simulink library "CTRL_LO_ST5"  (R2023b)
settings: Solver=VariableStepAuto  StartTime=0.0  StopTime=10.0  RelTol=1e-3
undefined symbols (not defined in the file): CTRL_LO_p_TqMotLoLim_Nm, CTRL_LO_p_TqMotUpLim_Nm, p_RadWhlDynFr_m, p_RadWhlDynRe_m, p_RatGearFr_na, p_trackFr_m, p_trackRe_m
libraries: slpidlib x4, simulink x1
settings Model: Creator=blatak  LastModifiedBy=blatak

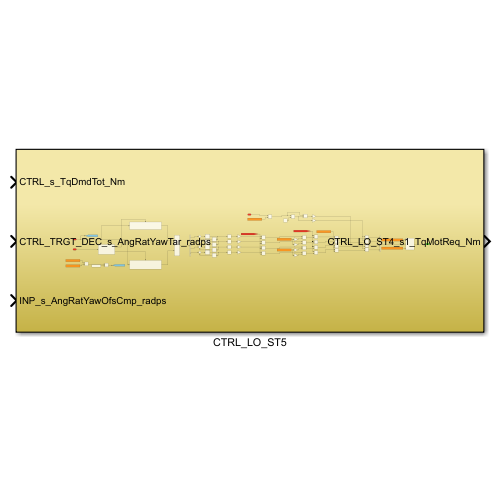
[thumbnail: Simulink's stored preview of the top-level diagram]
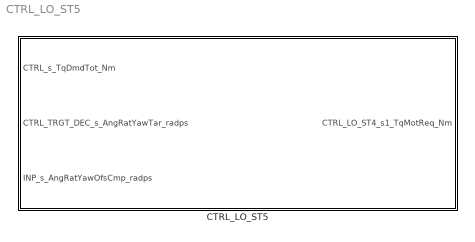
== system CTRL_LO_ST5 ==
  CTRL_LO_ST5 : Subsystem

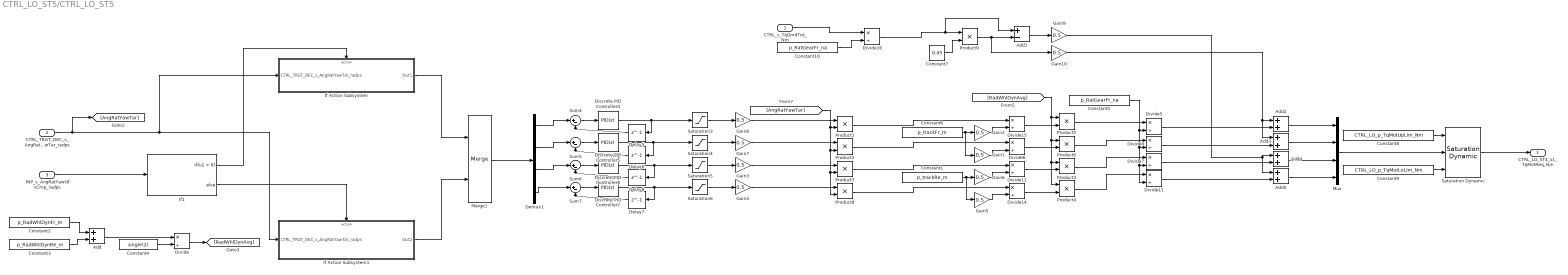
== system CTRL_LO_ST5/CTRL_LO_ST5 ==
  CTRL_s_TqDmdTot_Nm : Inport
  CTRL_TRGT_DEC_s_AngRatYawTar_radps : Inport  Port=2
  INP_s_AngRatYawOfsCmp_radps : Inport  Port=3
  Add{,2..5} (5 alike) : Sum
  Add1 : Sum  Inputs=+-
  Constant1 : Constant  Value=p_trackRe_m
  Constant10 : Constant  Value=p_RatGearFr_na
  Constant2 : Constant  Value=p_RadWhlDynFr_m
  Constant3 : Constant  Value=p_RadWhlDynRe_m
  Constant4 : Constant  Value=single(2)
  Constant5 : Constant  Value=p_RatGearFr_na
  Constant6 : Constant  Value=p_trackFr_m
  Constant7 : Constant  Value=0.45
  Constant8 : Constant  Value=CTRL_LO_p_TqMotUpLim_Nm
  Constant9 : Constant  Value=CTRL_LO_p_TqMotLoLim_Nm
  Delay{5..8} (4 alike) : Delay  DelayLength=1
  Demux1 : Demux
  Discrete PID Controller{4..7} (4 alike) : slpidlib/PID Controller  Controller=PID  Form=Parallel  TimeDomain=Discrete-time  UseExternalTs=off  SampleTime=-1  IntegratorMethod=Forward Euler  FilterMethod=Forward Euler  ControllerParametersSource=internal  P=0.1  I=10  UseKiTs=off  D=0  N=100  UseFilter=on  TunerSelectOption=Transfer Function Based (PID Tuner App)  InitialConditionSource=internal  InitialConditionForIntegrator=0  InitialConditionForFilter=0  DifferentiatorICPrevScaledInput=0  ExternalReset=none  TrackingMode=off  Kt=1  LimitOutput=off  SatLimitsSource=internal  UpperSaturationLimit=inf  LowerSaturationLimit=-inf  LinearizeAsGain=off  AntiWindupMode=none  Kb=1  LimitIntegrator=off  UpperIntegratorSaturationLimit=inf  LowerIntegratorSaturationLimit=-inf  POutMin=[]  POutMax=[]  IOutMin=[]  IOutMax=[]  DOutMin=[]  DOutMax=[]  NOutMin=[]  NOutMax=[]  SumOutMin=[]  SumOutMax=[]  SaturationOutMin=[]  SaturationOutMax=[]  PParamMin=[]  PParamMax=[]  IParamMin=[]  IParamMax=[]  DParamMin=[]  DParamMax=[]  NParamMin=[]  NParamMax=[]  KbParamMin=[]  KbParamMax=[]  KtParamMin=[]  KtParamMax=[]  KbOutMin=[]  KbOutMax=[]  KtOutMin=[]  KtOutMax=[]  IntegratorOutMin=[]  IntegratorOutMax=[]  FilterOutMin=[]  FilterOutMax=[]  SumI1OutMin=[]  SumI1OutMax=[]  SumI2OutMin=[]  SumI2OutMax=[]  SumI3OutMin=[]  SumI3OutMax=[]  SumI4OutMin=[]  SumI4OutMax=[]  SumDOutMin=[]  SumDOutMax=[]  DifferentiatorOutMin=[]  DifferentiatorOutMax=[]  FilterDiffOutCoefMin=[]  FilterDiffOutCoefMax=[]  ReciprocalOutMin=[]  ReciprocalOutMax=[]  SumDenOutMin=[]  SumDenOutMax=[]  SumNumOutMin=[]  SumNumOutMax=[]  DivideOutMin=[]  DivideOutMax=[]  UdiffTsProdOutMin=[]  UdiffTsProdOutMax=[]  NTsProdOutMin=[]  NTsProdOutMax=[]  UintegralTsProdOutMin=[]  UintegralTsProdOutMax=[]  UngainTsProdOutMin=[]  UngainTsProdOutMax=[]  ClampingZeroOutDataTypeStr=Inherit: Inherit via back propagation  ClampingZeroOutMin=[]  ClampingZeroOutMax=[]  FilterDenConstantOutDataTypeStr=Inherit: Inherit via back propagation  FilterDenConstantOutMin=[]  FilterDenConstantOutMax=[]  PCopyOutDataTypeStr=Inherit: Inherit via back propagation  PCopyOutMin=[]  PCopyOutMax=[]  NCopyOutDataTypeStr=Inherit: Inherit via back propagation  NCopyOutMin=[]  NCopyOutMax=[]  IntegratorContinuousStateAttributes=''  IntegratorStateMustResolveToSignalObject=off  IntegratorRTWStateStorageClass=Auto  FilterContinuousStateAttributes=''  FilterStateMustResolveToSignalObject=off  FilterRTWStateStorageClass=Auto  ParallelPVariant=InternalParameters  IdealPVariant=Disabled  IVariant=InternalParameters  DVariant=InternalParameters  IntegratorVariant=Discrete  SatVariant=Disabled  AWVariant=Passthrough  PCopyVariant=Disabled  TRVariant=Disabled  FdbkBlocksVariant=Forward  IdealPFdbkVariant=Disabled  SatFdbkVariant=Disabled  DerivativeFilterVariant=ForwardEulerFilter  NVariant=InternalParameters  NCopyVariant=Disabled  FilterICVariant=InternalICsFilter  IntegratorICVariant=InternalICs  ExternalResetVariant=Disabled  TRSumVariant=Passthrough  SumFdbkVariant=Disabled  SumVariant=Sum_PID  TsampFilterVariant=InternalTs  TsampNgainVariant=Passthrough  TsampIntegralVariant=Disabled_SignalSpec  ExternalSaturationOutDataTypeStr=Inherit: Same as second input
  Divide{,5..8,11..12,14..16} (10 alike) : Product  Inputs=*/
  Gain{1..10} (10 alike) : Gain  Gain=0.5
  If Action Subsystem : Subsystem  TreatAsAtomicUnit=on
  If Action Subsystem1 : Subsystem  TreatAsAtomicUnit=on
  If1 : If
  Merge1 : Merge
  Mux : Mux
  Product{1..9} (9 alike) : Product
  Saturation Dynamic : simulink/Discontinuities/Saturation Dynamic  OutMin=[]  OutMax=[]  OutDataTypeStr=Inherit: Same as second input  OutDataType=fixdt(1, 16)  OutScaling=2^-10  DoSatur=off
  Saturation{3..6} (4 alike) : Saturate  UpperLimit=1  LowerLimit=-1
  Sum{4..7} (4 alike) : Sum  Inputs=|+-
  CTRL_LO_ST4_s1_TqMotReq_Nm : Outport
  wires:
  Constant2/1 -> Add/1
  Constant3/1 -> Add/2
  Add/1 -> Divide/1
  Constant4/1 -> Divide/2
  CTRL_TRGT_DEC_s_AngRatYawTar_radps/1 -> [AngRatYawTar], If Action Subsystem/1(CTRL_TRGT_DEC_s_AngRatYawTar_radps), If Action Subsystem1/1(CTRL_TRGT_DEC_s_AngRatYawTar_radps)
  INP_s_AngRatYawOfsCmp_radps/1 -> If1/1
  If1/1 -> If Action Subsystem/Action
  If1/2 -> If Action Subsystem1/Action
  If Action Subsystem/1(Out1) -> Merge1/1
  If Action Subsystem1/1(Out2) -> Merge1/2
  Divide12/1 -> Product3/2
  Saturation4/1 -> Gain7/1
  Discrete PID Controller6/1 -> Saturation5/1, Delay8/1
  Product7/1 -> Divide12/1
  Demux1/2 -> Sum5/1
  Gain8/1 -> Product1/1
  Product6/1 -> Divide8/1
  Demux1/4 -> Sum7/1
  Gain6/1 -> Divide12/2
  Constant5/1 -> Divide7/2, Divide11/2, Divide8/2, Divide5/2
  Product1/1 -> Divide15/1
  Product2/1 -> Divide6/1
  Demux1/3 -> Sum6/1
  Product8/1 -> Divide14/1
  Saturation3/1 -> Gain8/1
  Gain1/1 -> Divide6/2
  Delay8/1 -> Sum6/2
  Discrete PID Controller5/1 -> Delay6/1, Saturation4/1
  [AngRatYawTar] -> Product7/2, Product8/2, Product2/2, Product1/2
  Discrete PID Controller4/1 -> Saturation3/1, Delay5/1
  Constant1/1 -> Gain5/1, Gain6/1
  Saturation5/1 -> Gain3/1
  Gain7/1 -> Product2/1
  Sum5/1 -> Discrete PID Controller5/1
  Divide6/1 -> Product6/2
  Discrete PID Controller7/1 -> Saturation6/1, Delay7/1
  Sum6/1 -> Discrete PID Controller6/1
  Gain4/1 -> Product8/1
  Demux1/1 -> Sum4/1
  Product5/1 -> Divide5/1
  Delay5/1 -> Sum4/2
  Product3/1 -> Divide7/1
  Product4/1 -> Divide11/1
  Gain2/1 -> Divide15/2
  Delay6/1 -> Sum5/2
  Gain5/1 -> Divide14/2
  Saturation6/1 -> Gain4/1
  Divide14/1 -> Product4/2
  Merge1/1 -> Demux1/1
  Constant6/1 -> Gain1/1, Gain2/1
  Sum7/1 -> Discrete PID Controller7/1
  Delay7/1 -> Sum7/2
  [RadWhlDynAvg] -> Product3/1, Product4/1, Product6/1, Product5/1
  Gain3/1 -> Product7/1
  Divide15/1 -> Product5/2
  Sum4/1 -> Discrete PID Controller4/1
  Divide/1 -> [RadWhlDynAvg]
  CTRL_s_TqDmdTot_Nm/1 -> Divide16/1
  Product9/1 -> Add1/2, Gain10/1
  Gain9/1 -> Add4/1, Add5/1
  Add1/1 -> Gain9/1
  Constant7/1 -> Product9/2
  Divide16/1 -> Product9/1, Add1/1
  Gain10/1 -> Add3/1, Add2/1
  Constant10/1 -> Divide16/2
  Divide5/1 -> Add2/2
  Divide8/1 -> Add3/2
  Divide7/1 -> Add4/2
  Divide11/1 -> Add5/2
  Add5/1 -> Mux/4
  Add4/1 -> Mux/3
  Add3/1 -> Mux/2
  Add2/1 -> Mux/1
  Constant8/1 -> Saturation Dynamic/1
  Constant9/1 -> Saturation Dynamic/3
  Mux/1 -> Saturation Dynamic/2
  Saturation Dynamic/1 -> CTRL_LO_ST4_s1_TqMotReq_Nm/1

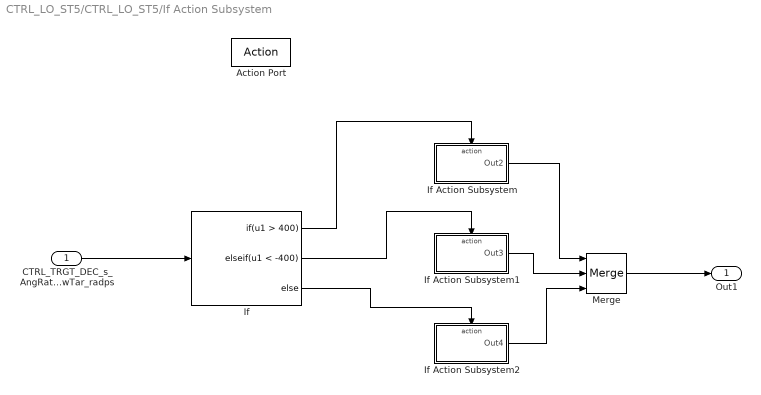
== system CTRL_LO_ST5/CTRL_LO_ST5/If Action Subsystem ==
  CTRL_TRGT_DEC_s_AngRatYawTar_radps : Inport
  Action Port : ActionPort  ActionPortLabel=if(u1 > 0)
  If : If  IfExpression=u1 > 400  ElseIfExpressions=u1 < -400
  If Action Subsystem : Subsystem  TreatAsAtomicUnit=on
  If Action Subsystem1 : Subsystem  TreatAsAtomicUnit=on
  If Action Subsystem2 : Subsystem  TreatAsAtomicUnit=on
  Merge : Merge  Inputs=3
  Out1 : Outport
  wires:
  If Action Subsystem2/1(Out4) -> Merge/3
  CTRL_TRGT_DEC_s_AngRatYawTar_radps/1 -> If/1
  If/2 -> If Action Subsystem1/Action
  If/1 -> If Action Subsystem/Action
  If Action Subsystem1/1(Out3) -> Merge/2
  If/3 -> If Action Subsystem2/Action
  Merge/1 -> Out1/1
  If Action Subsystem/1(Out2) -> Merge/1

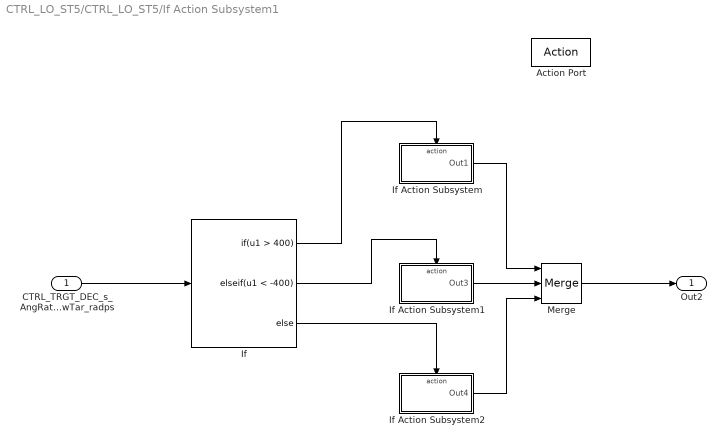
== system CTRL_LO_ST5/CTRL_LO_ST5/If Action Subsystem1 ==
  CTRL_TRGT_DEC_s_AngRatYawTar_radps : Inport
  Action Port : ActionPort  ActionPortLabel=else
  If : If  IfExpression=u1 > 400  ElseIfExpressions=u1 < -400
  If Action Subsystem : Subsystem  TreatAsAtomicUnit=on
  If Action Subsystem1 : Subsystem  TreatAsAtomicUnit=on
  If Action Subsystem2 : Subsystem  TreatAsAtomicUnit=on
  Merge : Merge  Inputs=3
  Out2 : Outport
  wires:
  If Action Subsystem2/1(Out4) -> Merge/3
  If Action Subsystem1/1(Out3) -> Merge/2
  If/1 -> If Action Subsystem/Action
  If/2 -> If Action Subsystem1/Action
  Merge/1 -> Out2/1
  If Action Subsystem/1(Out1) -> Merge/1
  If/3 -> If Action Subsystem2/Action
  CTRL_TRGT_DEC_s_AngRatYawTar_radps/1 -> If/1

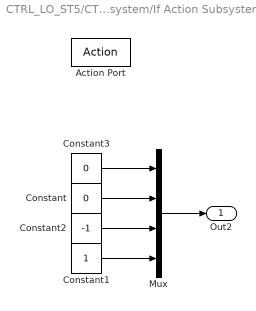
== system CTRL_LO_ST5/CTRL_LO_ST5/If Action Subsystem/If Action Subsystem ==
  Action Port : ActionPort  ActionPortLabel=if(u1 > 400)
  Constant : Constant  Value=0
  Constant1 : Constant
  Constant2 : Constant  Value=-1
  Constant3 : Constant  Value=0
  Mux : Mux
  Out2 : Outport
  wires:
  Mux/1 -> Out2/1
  Constant3/1 -> Mux/1
  Constant/1 -> Mux/2
  Constant2/1 -> Mux/3
  Constant1/1 -> Mux/4

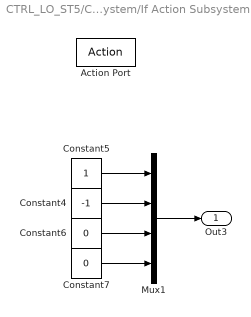
== system CTRL_LO_ST5/CTRL_LO_ST5/If Action Subsystem/If Action Subsystem1 ==
  Action Port : ActionPort  ActionPortLabel=elseif(u1 < -400)
  Constant4 : Constant  Value=-1
  Constant5 : Constant
  Constant6 : Constant  Value=0
  Constant7 : Constant  Value=0
  Mux1 : Mux
  Out3 : Outport
  wires:
  Constant7/1 -> Mux1/4
  Constant4/1 -> Mux1/2
  Constant5/1 -> Mux1/1
  Constant6/1 -> Mux1/3
  Mux1/1 -> Out3/1

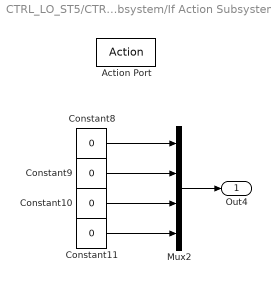
== system CTRL_LO_ST5/CTRL_LO_ST5/If Action Subsystem/If Action Subsystem2 ==
  Action Port : ActionPort  ActionPortLabel=else
  Constant{8..11} (4 alike) : Constant  Value=0
  Mux2 : Mux
  Out4 : Outport
  wires:
  Mux2/1 -> Out4/1
  Constant11/1 -> Mux2/4
  Constant10/1 -> Mux2/3
  Constant8/1 -> Mux2/1
  Constant9/1 -> Mux2/2

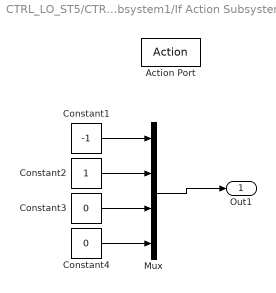
== system CTRL_LO_ST5/CTRL_LO_ST5/If Action Subsystem1/If Action Subsystem ==
  Action Port : ActionPort  ActionPortLabel=if(u1 > 400)
  Constant1 : Constant  Value=-1
  Constant2 : Constant
  Constant3 : Constant  Value=0
  Constant4 : Constant  Value=0
  Mux : Mux
  Out1 : Outport
  wires:
  Constant4/1 -> Mux/4
  Constant2/1 -> Mux/2
  Mux/1 -> Out1/1
  Constant1/1 -> Mux/1
  Constant3/1 -> Mux/3

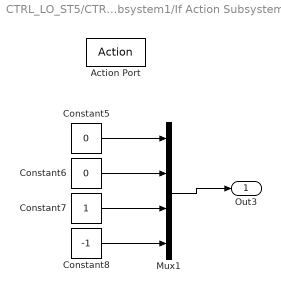
== system CTRL_LO_ST5/CTRL_LO_ST5/If Action Subsystem1/If Action Subsystem1 ==
  Action Port : ActionPort  ActionPortLabel=elseif(u1 < -400)
  Constant5 : Constant  Value=0
  Constant6 : Constant  Value=0
  Constant7 : Constant
  Constant8 : Constant  Value=-1
  Mux1 : Mux
  Out3 : Outport
  wires:
  Constant6/1 -> Mux1/2
  Constant8/1 -> Mux1/4
  Constant7/1 -> Mux1/3
  Constant5/1 -> Mux1/1
  Mux1/1 -> Out3/1

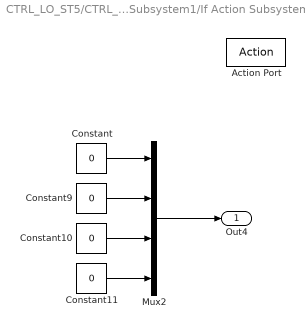
== system CTRL_LO_ST5/CTRL_LO_ST5/If Action Subsystem1/If Action Subsystem2 ==
  Action Port : ActionPort  ActionPortLabel=else
  Constant{,9..11} (4 alike) : Constant  Value=0
  Mux2 : Mux
  Out4 : Outport
  wires:
  Constant/1 -> Mux2/1
  Constant9/1 -> Mux2/2
  Mux2/1 -> Out4/1
  Constant10/1 -> Mux2/3
  Constant11/1 -> Mux2/4
